simulink model "plant_and_actuator"  (R2018a)
settings: Solver=FixedStepAuto  StartTime=0.0  StopTime=100  FixedStep=0.1  RelTol=1e-3
undefined symbols (not defined in the file): D, I, P
settings Model: Creator=Łukasz  LastModifiedBy=Łukasz
settings DataIOCC: SaveFormat=Structure  SignalLogging=off  DSMLogging=off

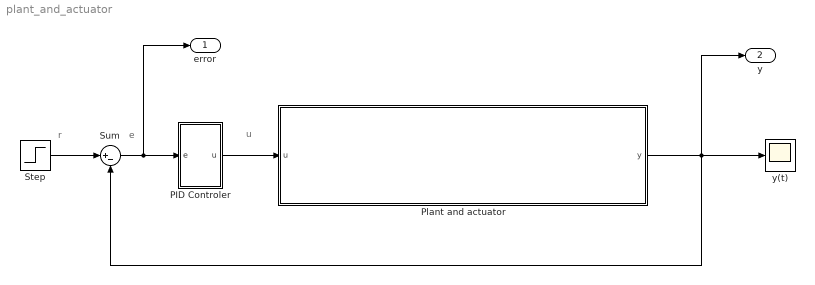
== system plant_and_actuator ==
  note: u
  note: r
  note: e
  PID Controler : Subsystem  mask{P=P, I=I, D=D}
      mask DialogControl DescGroupVar Prompt: PID Controler
      mask DialogControl DescTextVar Prompt: A proportional–integral–derivative controller
      mask DialogControl Control2 Prompt: Proportional gain
      mask DialogControl Control3 Prompt: Integral gain
      mask DialogControl Control4 Prompt: Derivative gain
  Plant and actuator : Subsystem
  Step : Step  SampleTime=0
  Sum : Sum  Inputs=|+-
  "y(t) " : Scope
  error : Outport
  y : Outport  Port=2
  wires:
  PID Controler/1(u) -> Plant and actuator/1(u)
  Sum/1 -> PID Controler/1(e), error/1
  Plant and actuator/1(y) -> y/1, "y(t) "/1, Sum/2
  Step/1 -> Sum/1

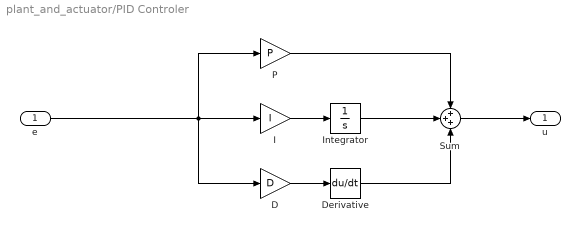
== system plant_and_actuator/PID Controler ==
  e : Inport
  D : Gain  Gain=D
  Derivative : Derivative
  I : Gain  Gain=I
  Integrator : Integrator
  P : Gain  Gain=P
  Sum : Sum  Inputs=+++
  u : Outport
  wires:
  D/1 -> Derivative/1
  e/1 -> D/1, P/1, I/1
  I/1 -> Integrator/1
  Integrator/1 -> Sum/2
  Derivative/1 -> Sum/3
  P/1 -> Sum/1
  Sum/1 -> u/1

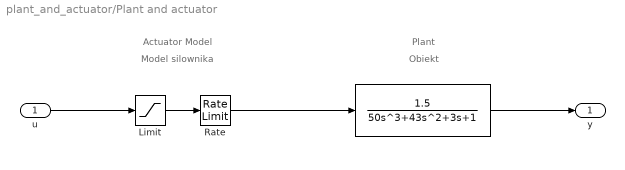
== system plant_and_actuator/Plant and actuator ==
  note: Obiekt
  note: Model silownika
  note: Plant
  note: Actuator Model
  u : Inport
  " " : TransferFcn  Numerator=[1.5]  Denominator=[50 43 3 1]
  Limit : Saturate  UpperLimit=2  LowerLimit=-2
  Rate : RateLimiter  RisingSlewLimit=0.8  FallingSlewLimit=-0.8  SampleTimeMode=inherited
  y : Outport
  wires:
  u/1 -> Limit/1
  Rate/1 -> " "/1
  " "/1 -> y/1
  Limit/1 -> Rate/1
